simulink model "DistributionFlow"  (R2023b)
settings: Solver=FixedStepDiscrete  StartTime=0.0  StopTime=30  RelTol=1e-3
libraries: moneylib x5, simulink x2
settings Model: Creator=gcampa  LastModifiedBy=gcampa
settings SolverCC: AlgebraicLoopSolver=TrustRegion
settings DataIOCC: SaveFormat=Array  SignalLogging=off  DSMLogging=off  SaveTime=off
settings OptimizationCC: ReuseModelBlockBuffer=off
settings DebuggingCC: UnconnectedInputMsg=warning  UnconnectedOutputMsg=warning  UnconnectedLineMsg=warning
settings ModelReferenceCC: EnableRefExpFcnMdlSchedulingChecks=on
settings RTWCC: DLArmComputeVersion=19.05

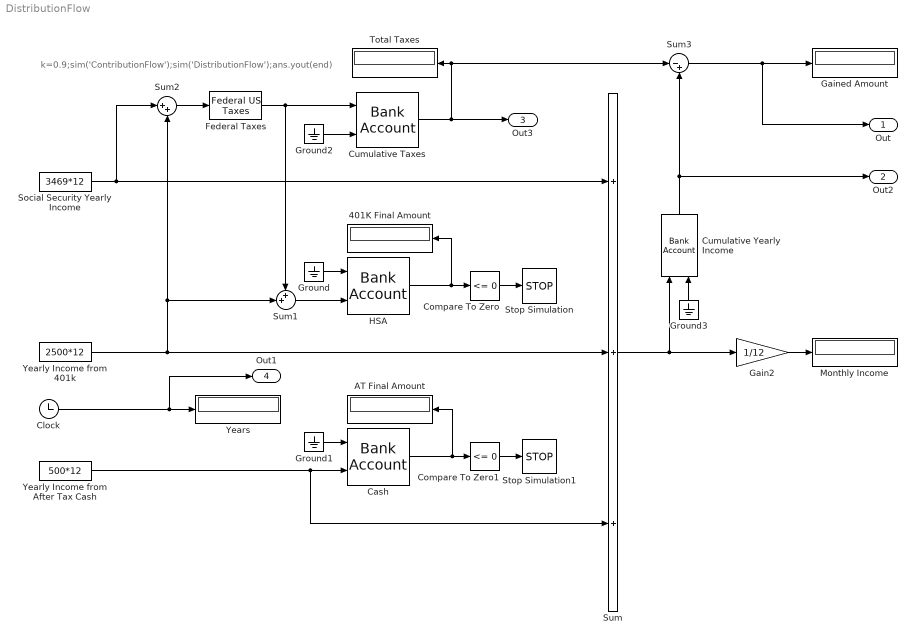
== system DistributionFlow ==
  note: k=0.9;sim('ContributionFlow');sim('DistributionFlow');ans.yout(end)
  401K Final Amount : Display
      settings: Format=bank
  AT Final Amount : Display
      settings: Format=bank
  Cash : moneylib/Bank Account  i=0.01  j=0.03  x0=Cash
  Clock : Clock
  Compare To Zero : simulink/Logic and Bit Operations/Compare To Zero  relop=<=  OutDataTypeStr=boolean
  Compare To Zero1 : simulink/Logic and Bit Operations/Compare To Zero  relop=<=  OutDataTypeStr=boolean
  Cumulative Yearly Income : moneylib/Bank Account  i=0  j=0  x0=0
  Cumulative Taxes : moneylib/Bank Account  i=0  j=0  x0=Taxes
  Federal Taxes : moneylib/Federal US Taxes  x=[9875 40125 85525 163300 207350 518400]  p=[0.10 0.12 0.22 0.24 0.32 0.35 0.37]
  Gain2 : Gain  Gain=1/12
  Gained Amount : Display
      settings: Format=bank
  Ground{,1..3} (4 alike) : Ground
  HSA : moneylib/Bank Account  i=0.01  j=0.03  x0=Taxable
  Monthly Income : Display
      settings: Format=bank
  Social Security Yearly Income : Constant  Value=3469*12
  Stop Simulation : Stop
  Stop Simulation1 : Stop
  Sum : Sum  Inputs=+++
  Sum1 : Sum  Inputs=++|
  Sum2 : Sum  Inputs=|++
  Sum3 : Sum  Inputs=|-+
  Total Taxes : Display
      settings: Format=bank
  Yearly Income from 401k : Constant  Value=2500*12
  Yearly Income from After Tax Cash : Constant  Value=500*12
  Years : Display
      settings: Format=bank
  Out : Outport
  Out2 : Outport  Port=2
  Out3 : Outport  Port=3
  Out1 : Outport  Port=4
  wires:
  Ground/1 -> HSA/1
  Ground1/1 -> Cash/1
  HSA/1 -> Compare To Zero/1, 401K Final Amount/1
  Yearly Income from After Tax Cash/1 -> Cash/2, Sum/3
  Sum/1 -> Cumulative Yearly Income/1, Gain2/1
  Federal Taxes/1 -> Cumulative Taxes/1, Sum1/1
  Clock/1 -> Out1/1, Years/1
  Compare To Zero/1 -> Stop Simulation/1
  Cash/1 -> AT Final Amount/1, Compare To Zero1/1
  Compare To Zero1/1 -> Stop Simulation1/1
  Ground2/1 -> Cumulative Taxes/2
  Cumulative Taxes/1 -> Sum3/1, Total Taxes/1, Out3/1
  Ground3/1 -> Cumulative Yearly Income/2
  Sum1/1 -> HSA/2
  Gain2/1 -> Monthly Income/1
  Yearly Income from 401k/1 -> Sum/2, Sum2/2, Sum1/2
  Social Security Yearly Income/1 -> Sum2/1, Sum/1
  Sum2/1 -> Federal Taxes/1
  Cumulative Yearly Income/1 -> Out2/1, Sum3/2
  Sum3/1 -> Out/1, Gained Amount/1
